simulink model "tank_sf_nozerocross"  (Simulink 4.00)
settings: Solver=ode45  StartTime=0.0  StopTime=10.0  RelTol=1e-3
settings Model: LastModifiedBy=hespanha  BlockReductionOpt=off

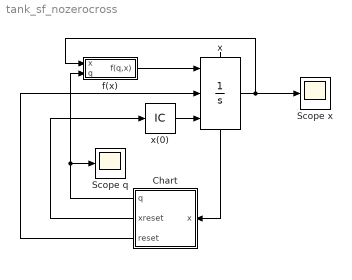
== system tank_sf_nozerocross ==
  Chart : Stateflow chart  Orientation=left
      settings: RTWFcnNameOpts=Auto  RTWFileNameOpts=Auto
  Scope q : Scope
      settings: TimeRange=10  YMin=0  YMax=5  SaveToWorkspace=off  LimitDataPoints=on  MaxDataPoints=5000
  Scope x : Scope
      settings: TimeRange=10  YMin=-1  YMax=5  SaveToWorkspace=off  SaveName=ScopeData  LimitDataPoints=on  MaxDataPoints=5000
  f(x) : Subsystem  Description=f(x)
      settings: RTWFcnNameOpts=Auto  RTWFileNameOpts=Auto
  x : Integrator  ExternalReset=either  InitialConditionSource=external  InitialCondition=0  LimitOutput=off  UpperSaturationLimit=inf  LowerSaturationLimit=-inf  ShowSaturationPort=off  ShowStatePort=on  AbsoluteTolerance=auto
  x(0) : InitialCondition  Value=[4;0]
  wires:
  x(0)/1 -> x/3
  f(x)/1(f(q,x)) -> x/1
  x/1 -> Scope x/1, f(x)/1(x)
  Chart/1(q) -> Scope q/1, f(x)/2(q)
  Chart/3(reset) -> x/2
  Chart/2(xreset) -> x(0)/1
  x/State -> Chart/1(x)

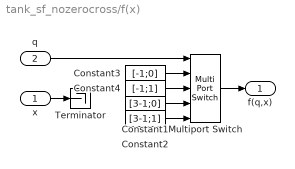
== system tank_sf_nozerocross/f(x) ==
  x : Inport  Port=1
  q : Inport  Port=2
  Constant1 : Constant  Value=[3-1;0]
  Constant2 : Constant  Value=[3-1;1]
  Constant3 : Constant  Value=[-1;0]
  Constant4 : Constant  Value=[-1;1]
  Multiport Switch : MultiPortSwitch  Inputs=4
  Terminator : Terminator
  f(q,x) : Outport  Port=1
  wires:
  q/1 -> Multiport Switch/1
  Constant3/1 -> Multiport Switch/2
  Multiport Switch/1 -> f(q,x)/1
  Constant4/1 -> Multiport Switch/3
  Constant1/1 -> Multiport Switch/4
  Constant2/1 -> Multiport Switch/5
  x/1 -> Terminator/1

== stateflow chart Chart ==
  state pump_off/
    entry:q=1;
  state wait_to_on/
    entry:q=2;
  state pump_on/
    entry:q=3;
  state wait_to_off/
    entry:q=4;
  wait_to_off -> pump_off : [x[2]>=.5]
  (default) -> pump_off
  wait_to_on -> pump_on : [x[2]>=.5]
  pump_on -> wait_to_off : [x[1]>=2]/
      |   xreset[1]=x[1];
      |   xreset[2]=0;reset;
  pump_off -> wait_to_on : [x[1]<=1]/
      |   xreset[1]=x[1];
      |   xreset[2]=0;reset;
  data: q output int8 [1..4]; x input double size=2; xreset output double size=2
  events: reset output EITHER_EDGE_EVENT
